simulink model "sys2"  (R2022a)
settings: Solver=VariableStepAuto  StartTime=0.0  StopTime=30  RelTol=1e-3
values from neighbouring files (symbols this model uses):
  k = 1    [sys2m.m]    (also in sys3m.m = 0.5)
settings Model: Creator=Reizinho  LastModifiedBy=Reizinho

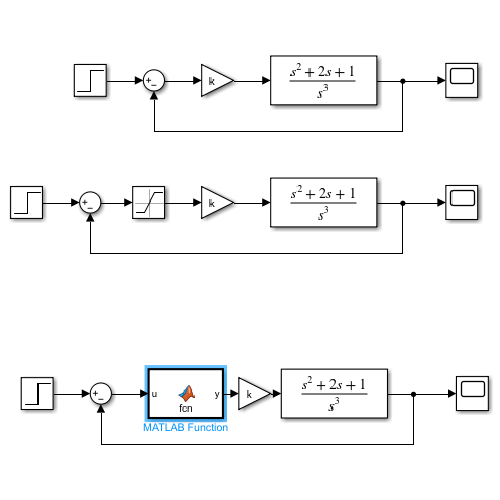
[thumbnail: Simulink's stored preview of the top-level diagram]
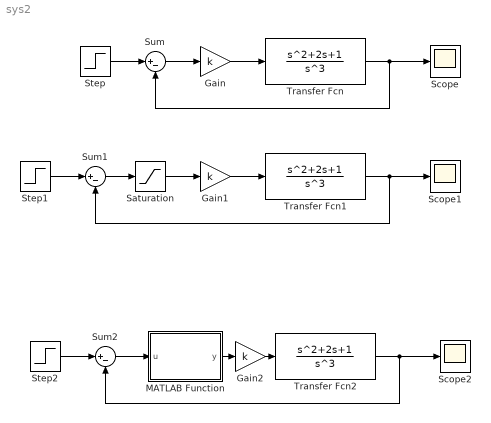
== system sys2 ==
  Gain : Gain  Gain=k
  Gain1 : Gain  Gain=k
  Gain2 : Gain  Gain=k
  MATLAB Function : MATLAB Function  TreatAsAtomicUnit=on
  Saturation : Saturate  UpperLimit=1  LowerLimit=-1
  Scope : Scope
  Scope1 : Scope
  Scope2 : Scope
  Step : Step  After=0.01  SampleTime=0.1
  Step1 : Step  After=4  SampleTime=0.1
  Step2 : Step  After=4  SampleTime=0.1
  Sum : Sum  Inputs=|+-
  Sum1 : Sum  Inputs=|+-
  Sum2 : Sum  Inputs=|+-
  Transfer Fcn : TransferFcn  Numerator=[1 2 1]  Denominator=[1 0 0 0]
  Transfer Fcn1 : TransferFcn  Numerator=[1 2 1]  Denominator=[1 0 0 0]
  Transfer Fcn2 : TransferFcn  Numerator=[1 2 1]  Denominator=[1 0 0 0]
  wires:
  Gain/1 -> Transfer Fcn/1
  Sum/1 -> Gain/1
  Transfer Fcn/1 -> Scope/1, Sum/2
  Step/1 -> Sum/1
  Step1/1 -> Sum1/1
  Transfer Fcn1/1 -> Scope1/1, Sum1/2
  Gain1/1 -> Transfer Fcn1/1
  Saturation/1 -> Gain1/1
  Sum1/1 -> Saturation/1
  Gain2/1 -> Transfer Fcn2/1
  Step2/1 -> Sum2/1
  Transfer Fcn2/1 -> Scope2/1, Sum2/2
  MATLAB Function/1(y) -> Gain2/1
  Sum2/1 -> MATLAB Function/1(u)

== matlab function sys2/MATLAB Function ==
  data: u input; y output
function y = fcn(u)

y = tanh(u/0.05);
